simulink model "powerwindow02"  (Simulink 6.0)
settings: Solver=ode23t  StartTime=0.0  StopTime=inf  FixedStep=1e-4  RelTol=1e-2
libraries: powerlib2 x22, mblibv1 x18, simulink x6
settings Model: Creator=The MathWorks Inc.  LastModifiedBy=batserve  ExtModeAutoUpdateStatusClock=off
settings DataIOCC: SignalLoggingName=sigsOut
settings OptimizationCC: BooleanDataType=off
settings DebuggingCC: CheckExecutionContextPreStartOutputMsg=on  CheckExecutionContextRuntimeOutputMsg=on  SolverPrmCheckMsg=none
settings HardwareCC: TargetUnknown=on
settings SimMechanicsCC: VisOnUpdateDiagram=on

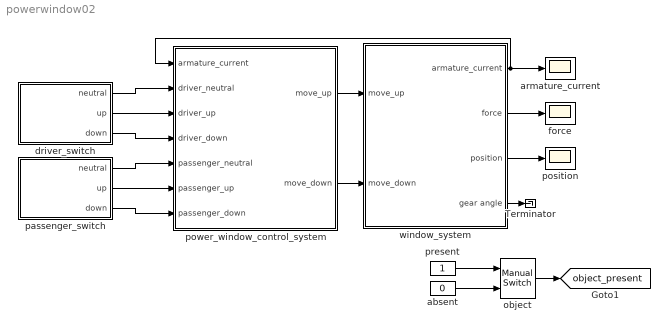
== system powerwindow02 ==
  Terminator : Terminator
  absent : Constant  Value=0
  armature_current : Scope
      settings: DataFormat=Array
  driver_switch : Subsystem  PropExecContextAcrossSSBoundary=on
  force : Scope
      settings: DataFormat=Array
  object : simulink/Signal Routing/Manual Switch  sw=1  action=0
  passenger_switch : Subsystem  PropExecContextAcrossSSBoundary=on
  position : Scope
      settings: YMin=-0.05  YMax=0.5  DataFormat=Array
  power_window_control_system : Subsystem  PropExecContextAcrossSSBoundary=on
  present : Constant
  window_system : Subsystem  PropExecContextAcrossSSBoundary=on
  tag scope: object_present=global
  wires:
  driver_switch/1(neutral) -> power_window_control_system/2(driver_neutral)
  driver_switch/2(up) -> power_window_control_system/3(driver_up)
  driver_switch/3(down) -> power_window_control_system/4(driver_down)
  passenger_switch/1(neutral) -> power_window_control_system/5(passenger_neutral)
  passenger_switch/2(up) -> power_window_control_system/6(passenger_up)
  passenger_switch/3(down) -> power_window_control_system/7(passenger_down)
  power_window_control_system/1(move_up) -> window_system/1(move_up)
  power_window_control_system/2(move_down) -> window_system/2(move_down)
  window_system/1(armature_current) -> armature_current/1, power_window_control_system/1(armature_current)
  window_system/2(force) -> force/1
  window_system/3(position) -> position/1
  present/1 -> object/1
  absent/1 -> object/2
  object/1 -> [object_present]
  window_system/4(gear angle) -> Terminator/1

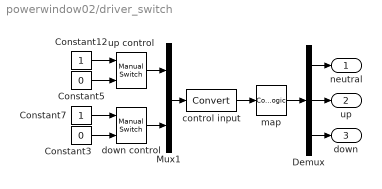
== system powerwindow02/driver_switch ==
  Constant12 : Constant
  Constant3 : Constant  Value=0
  Constant5 : Constant  Value=0
  Constant7 : Constant
  Demux : Demux  Outputs=3
  Mux1 : Mux  Inputs=2
  control input : DataTypeConversion  OutDataTypeMode=boolean  SaturateOnIntegerOverflow=on  RndMeth=Zero
  down control : simulink/Signal Routing/Manual Switch  sw=0  action=0
  map : CombinatorialLogic  TruthTable=[1 0 0;0 0 1;0 1 0;1 0 0]
  up control : simulink/Signal Routing/Manual Switch  sw=0  action=0
  neutral : Outport
  up : Outport  Port=2
  down : Outport  Port=3
  wires:
  control input/1 -> map/1
  Constant12/1 -> up control/1
  Constant5/1 -> up control/2
  Constant7/1 -> down control/1
  Constant3/1 -> down control/2
  down control/1 -> Mux1/2
  Mux1/1 -> control input/1
  up control/1 -> Mux1/1
  map/1 -> Demux/1
  Demux/1 -> neutral/1
  Demux/2 -> up/1
  Demux/3 -> down/1

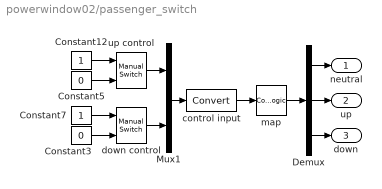
== system powerwindow02/passenger_switch ==
  Constant12 : Constant
  Constant3 : Constant  Value=0
  Constant5 : Constant  Value=0
  Constant7 : Constant
  Demux : Demux  Outputs=3
  Mux1 : Mux  Inputs=2
  control input : DataTypeConversion  OutDataTypeMode=boolean  SaturateOnIntegerOverflow=on  RndMeth=Zero
  down control : simulink/Signal Routing/Manual Switch  sw=0  action=0
  map : CombinatorialLogic  TruthTable=[1 0 0;0 0 1;0 1 0;1 0 0]
  up control : simulink/Signal Routing/Manual Switch  sw=0  action=0
  neutral : Outport
  up : Outport  Port=2
  down : Outport  Port=3
  wires:
  Demux/3 -> down/1
  Demux/2 -> up/1
  Demux/1 -> neutral/1
  map/1 -> Demux/1
  up control/1 -> Mux1/1
  Mux1/1 -> control input/1
  down control/1 -> Mux1/2
  Constant3/1 -> down control/2
  Constant7/1 -> down control/1
  Constant5/1 -> up control/2
  Constant12/1 -> up control/1
  control input/1 -> map/1

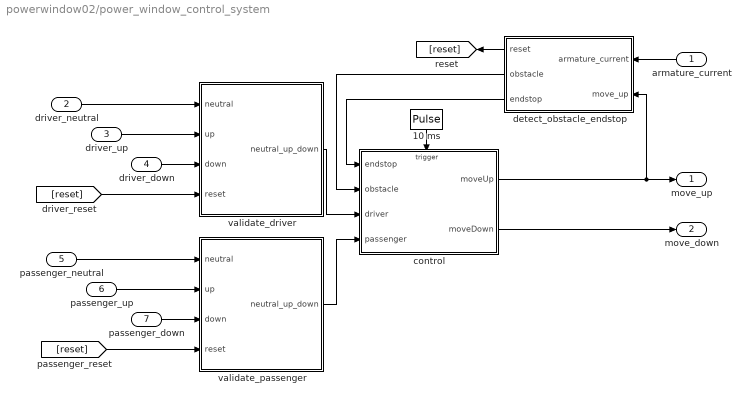
== system powerwindow02/power_window_control_system ==
  armature_current : Inport  Orientation=left  Port=1  LatchInput=off
  driver_neutral : Inport  Port=2  LatchInput=off
  driver_up : Inport  Port=3  LatchInput=off
  driver_down : Inport  Port=4  LatchInput=off
  passenger_neutral : Inport  Port=5  LatchInput=off
  passenger_up : Inport  Port=6  LatchInput=off
  passenger_down : Inport  Port=7  LatchInput=off
  10 ms : DiscretePulseGenerator  Orientation=down  SampleTime=10e-3
  control : Stateflow chart  TreatAsAtomicUnit=on  PropExecContextAcrossSSBoundary=on
  detect_obstacle_endstop : Subsystem  Orientation=left  PropExecContextAcrossSSBoundary=on
  validate_driver : Subsystem  PropExecContextAcrossSSBoundary=on
  validate_passenger : Subsystem  PropExecContextAcrossSSBoundary=on
  move_up : Outport
  move_down : Outport  Port=2
  wires:
  detect_obstacle_endstop/2(obstacle) -> control/2(obstacle)
  detect_obstacle_endstop/3(endstop) -> control/1(endstop)
  detect_obstacle_endstop/1(reset) -> [reset]
  armature_current/1 -> detect_obstacle_endstop/1(armature_current)
  10 ms/1 -> control/Trigger
  control/1(moveUp) -> detect_obstacle_endstop/2(move_up), move_up/1
  control/2(moveDown) -> move_down/1
  driver_neutral/1 -> validate_driver/1(neutral)
  driver_up/1 -> validate_driver/2(up)
  driver_down/1 -> validate_driver/3(down)
  [reset] -> validate_driver/4(reset)
  passenger_neutral/1 -> validate_passenger/1(neutral)
  passenger_up/1 -> validate_passenger/2(up)
  passenger_down/1 -> validate_passenger/3(down)
  [reset] -> validate_passenger/4(reset)
  validate_driver/1(neutral_up_down) -> control/3(driver)
  validate_passenger/1(neutral_up_down) -> control/4(passenger)

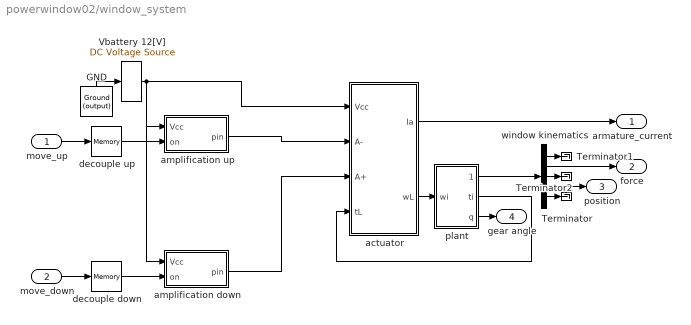
== system powerwindow02/window_system ==
  move_up : Inport  Port=1  LatchInput=off
  move_down : Inport  Port=2  LatchInput=off
  GND : powerlib2/Connectors/Ground (output)  Tag=PoWeRsYsTeMbLoCk  Orientation=up  PSBOutputType=1
  Terminator : Terminator
  Terminator1 : Terminator
  Terminator2 : Terminator
  Vbattery 12[V] : powerlib2/Electrical Sources/DC Voltage Source  Tag=PoWeRsYsTeMbLoCk  V=12  mesure=None  PSBOutputType=1
  actuator : Subsystem  PropExecContextAcrossSSBoundary=on
  amplification down : Subsystem  PropExecContextAcrossSSBoundary=on
  amplification up : Subsystem  PropExecContextAcrossSSBoundary=on
  decouple down : Memory
  decouple up : Memory
  plant : Subsystem  PropExecContextAcrossSSBoundary=on
  window kinematics : Demux  Outputs=[1,1,2,1,4]
  armature_current : Outport
  force : Outport  Port=2
  position : Outport  Port=3
  gear angle : Outport  Port=4
  wires:
  decouple down/1 -> amplification down/2(on)
  decouple up/1 -> amplification up/2(on)
  plant/3(q) -> gear angle/1
  GND/1 -> Vbattery 12[V]/1
  Vbattery 12[V]/1 -> amplification up/1(Vcc), amplification down/1(Vcc), actuator/1(Vcc)
  amplification up/1(pin) -> actuator/2(A-)
  amplification down/1(pin) -> actuator/3(A+)
  actuator/2(wL) -> plant/1(wi)
  plant/2(ti) -> actuator/4(tL)
  plant/1("F, x, v") -> window kinematics/1
  actuator/1(Ia) -> armature_current/1
  move_up/1 -> decouple up/1
  move_down/1 -> decouple down/1
  window kinematics/2 -> force/1
  window kinematics/1 -> Terminator1/1
  window kinematics/4 -> position/1
  window kinematics/5 -> Terminator/1
  window kinematics/3 -> Terminator2/1

== system powerwindow02/power_window_control_system/detect_obstacle_endstop ==
  armature_current : Inport  Port=1  LatchInput=off
  move_up : Inport  Port=2  LatchInput=off
  detect_endstop : Subsystem  PropExecContextAcrossSSBoundary=on
  detect_obstacle : Subsystem  PropExecContextAcrossSSBoundary=on
  either : Logic  Operator=OR
  process_current : Subsystem  PropExecContextAcrossSSBoundary=on
  reset : Outport
  obstacle : Outport  Port=2
  endstop : Outport  Port=3
  wires:
  armature_current/1 -> process_current/1(raw_current)
  detect_obstacle/1(obstacle) -> either/1, obstacle/1
  detect_endstop/1(endstop) -> endstop/1, either/2
  either/1 -> reset/1
  move_up/1 -> detect_obstacle/1(move_up)
  process_current/1(processed_current) -> detect_obstacle/2(armature_current), detect_endstop/1(armature_current)

== system powerwindow02/power_window_control_system/validate_driver ==
  neutral : Inport  Port=1  LatchInput=off
  up : Inport  Port=2  LatchInput=off
  down : Inport  Port=3  LatchInput=off
  reset : Inport  Port=4  LatchInput=off
  Mux : Mux  Inputs=3
  check_down : Subsystem  PropExecContextAcrossSSBoundary=on
  check_up : Subsystem  PropExecContextAcrossSSBoundary=on
  mutually_exclusive : Subsystem  PropExecContextAcrossSSBoundary=on
  neutral_up_down : Outport
  wires:
  Mux/1 -> neutral_up_down/1
  reset/1 -> [reset]
  [reset] -> check_down/2(reset)
  [reset] -> check_up/2(reset)
  check_up/1(checked_action) -> mutually_exclusive/2(up)
  neutral/1 -> mutually_exclusive/1(neutral)
  up/1 -> check_up/1(action)
  down/1 -> check_down/1(action)
  mutually_exclusive/1(validated_neutral) -> Mux/1
  mutually_exclusive/2(validated_up) -> Mux/2
  mutually_exclusive/3(validated_down) -> Mux/3
  check_down/1(checked_action) -> mutually_exclusive/3(down)

== system powerwindow02/power_window_control_system/validate_passenger ==
  neutral : Inport  Port=1  LatchInput=off
  up : Inport  Port=2  LatchInput=off
  down : Inport  Port=3  LatchInput=off
  reset : Inport  Port=4  LatchInput=off
  Mux : Mux  Inputs=3
  check_down : Subsystem  PropExecContextAcrossSSBoundary=on
  check_up : Subsystem  PropExecContextAcrossSSBoundary=on
  mutually_exclusive : Subsystem  PropExecContextAcrossSSBoundary=on
  neutral_up_down : Outport
  wires:
  Mux/1 -> neutral_up_down/1
  reset/1 -> [reset]
  [reset] -> check_down/2(reset)
  [reset] -> check_up/2(reset)
  check_up/1(checked_action) -> mutually_exclusive/2(up)
  neutral/1 -> mutually_exclusive/1(neutral)
  up/1 -> check_up/1(action)
  down/1 -> check_down/1(action)
  mutually_exclusive/1(validated_neutral) -> Mux/1
  mutually_exclusive/2(validated_up) -> Mux/2
  mutually_exclusive/3(validated_down) -> Mux/3
  check_down/1(checked_action) -> mutually_exclusive/3(down)

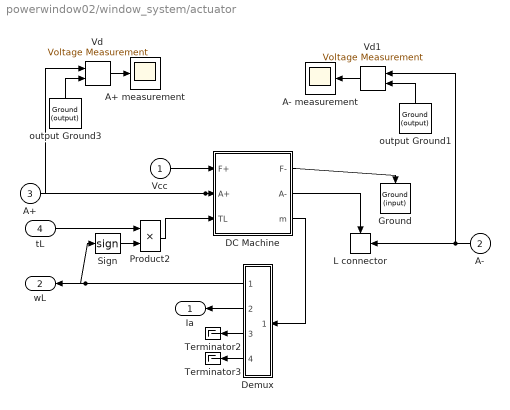
== system powerwindow02/window_system/actuator ==
  Vcc : Inport  Port=1  LatchInput=off
  A- : Inport  Orientation=left  Port=2  LatchInput=off
  A+ : Inport  Port=3  LatchInput=off
  tL : Inport  Port=4  LatchInput=off
  A+ measurement : Scope
      settings: TimeRange=0.12  YMin=11.8065  YMax=11.8095  SaveName=ScopeData2
  A- measurement : Scope
      settings: TimeRange=0.12  YMin=11.9431  YMax=11.9433  SaveName=ScopeData3
  DC Machine : Subsystem  PropExecContextAcrossSSBoundary=on  mask(DC machine){RLa=[0.15  0.036], RLf=[1.5 3], Laf=1, J=0.085, Bm=5, Tf=0, w0=0, PSBOutputType=110}
      mask prompts: RLa "Armature resistance and inductance [Ra (ohms) La (H) ]"; RLf "Field resistance and inductance [Rf (ohms) Lf (H) ]"; Laf "Field-armature mutual inductance Laf (H) :"; J "Total inertia J (kg.m^2)"; Bm "Viscous friction coefficient Bm (N.m.s)"; Tf "Coulomb friction torque Tf (N.m)"; w0 "Initial speed (rad/s) :"; PSBOutputType "Output type"
      mask help:
      | This block implements a separately excited DC machine. Access is provided  to the field connections so that the machine can be used as a shunt-connected or a series-connected  DC machine.
      |
      | Input 1 and output 1 : positive and negative armature terminals
      | Input 2 and output 2 : positive and negative field terminals
      | Input 3    : Load torque
      | Output 3 : Simulink measurement output [ w Ia If Te ]
      mask init:
      | Ra=RLa(1); La=RLa(2);
      | Rf=RLf(1); Lf=RLf(2);
      mask Help: web(psbhelp)
      mask Display: plot(-80,-80,80,80,[0,9,18,24,29,30,29,24,18,9,0,-9,-18,-24,-29,-30,-29,-24,-18,-9,0],[30,29,24,18,9,0,-9,-18,-24,-29,-30,-29,-24,-18,-9,0,9,18,24,29,30],[-29,-35,-35,-29],[-8,-8,8,8],[29,35,35,29],[-8,-8,8,8],[-35,-55],[0,0],[35,55],[0,0],[-78,-50,-50,-49,-45,-39,-33,-26,-21,-18,-17,-19,-22,-22,-26,-27,-25,-22,-16,-9,-3,2,6,6,4,1,1,-3,-4,-2,2,7,14,20,26,29,30,28,24,24,21,20,21,25,31,37,44,49,50,50,50,78]*.7,[58,58,57.2,49.2,42.8,38.8,38,39.6,44.4,51.6,59.6,67.6,72.4,72.4,65.2,57.2,49.2,42.8,38.8,38,39.6,44.4,51.6,59.6,67.6,72.4,72.4,65.2,57.2,49.2,42.8,38.8,38,39.6,44.4,51.6,59.6,67.6,72.4,72.4,65.2,57.2,49.2,42.8,38.8,38,39.6,44.4,51.6,58,58,58]*.6+15 );
  Demux : Subsystem  Orientation=left  PropExecContextAcrossSSBoundary=on
  Ground : powerlib2/Connectors/Ground (input)  Tag=PoWeRsYsTeMbLoCk  Orientation=down
  L connector : powerlib2/Connectors/L connector  Tag=PoWeRsYsTeMbLoCk  Orientation=left
  Product2 : Product  SaturateOnIntegerOverflow=on  InputSameDT=on
  Sign : Signum
  Terminator2 : Terminator
  Terminator3 : Terminator
  Vd : powerlib2/Measurements/Voltage Measurement  Tag=PoWeRsYsTeMmEaSuReMeNt  PhasorSimulation=off  OutputType=Magnitude  PSBOutputType=0  PSBequivalent=0
  Vd1 : powerlib2/Measurements/Voltage Measurement  Tag=PoWeRsYsTeMmEaSuReMeNt  Orientation=left  PhasorSimulation=off  OutputType=Magnitude  PSBOutputType=0  PSBequivalent=0
  output Ground1 : powerlib2/Connectors/Ground (output)  Tag=PoWeRsYsTeMbLoCk  Orientation=up  PSBOutputType=1
  output Ground3 : powerlib2/Connectors/Ground (output)  Tag=PoWeRsYsTeMbLoCk  Orientation=up  PSBOutputType=1
  Ia : Outport  Orientation=left
  wL : Outport  Orientation=left  Port=2
  wires:
  A+/1 -> DC Machine/2(A+), Vd/1
  Demux/4(Te) -> Terminator3/1
  Demux/3(If) -> Terminator2/1
  DC Machine/3(m) -> Demux/1(m)
  Demux/1(wm) -> Sign/1, wL/1
  Sign/1 -> Product2/2
  Product2/1 -> DC Machine/3(TL)
  tL/1 -> Product2/1
  Demux/2(Ia) -> Ia/1
  DC Machine/1(F-) -> Ground/1
  Vcc/1 -> DC Machine/1(F+)
  A-/1 -> Vd1/1, L connector/1
  DC Machine/2(A-) -> L connector/Enable
  output Ground3/1 -> Vd/2
  Vd/1 -> A+ measurement/1
  output Ground1/1 -> Vd1/2
  Vd1/1 -> A- measurement/1

== system powerwindow02/window_system/amplification down ==
  Vcc : Inport  Port=1  LatchInput=off
  on : Inport  Port=2  LatchInput=off
  Logical Operator : Logic  Operator=NOT
  Terminator1 : Terminator
  Terminator2 : Terminator
  connector : powerlib2/Connectors/T connector  Tag=PoWeRsYsTeMbLoCk  PSBOutputType=1
  output Ground1 : powerlib2/Connectors/Ground (output)  Tag=PoWeRsYsTeMbLoCk  Orientation=up  PSBOutputType=1
  up switch : powerlib2/Power Electronics/Ideal Switch  Tag=PoWeRsYsTeMbLoCk  Ron=0.01  Lon=0  IC=0  Rs=1000000  Cs=inf  PSBOutputType=10
  up switch1 : powerlib2/Power Electronics/Ideal Switch  Tag=PoWeRsYsTeMbLoCk  Ron=0.01  Lon=0  IC=0  Rs=1000000  Cs=inf  PSBOutputType=10
  pin : Outport  InitialOutput=0
  wires:
  on/1 -> Logical Operator/1, up switch/2
  Vcc/1 -> up switch/1
  up switch/2 -> Terminator1/1
  output Ground1/1 -> up switch1/1
  up switch1/2 -> Terminator2/1
  up switch/1 -> connector/1
  connector/1 -> pin/1
  up switch1/1 -> connector/Enable
  Logical Operator/1 -> up switch1/2

== system powerwindow02/window_system/amplification up ==
  Vcc : Inport  Port=1  LatchInput=off
  on : Inport  Port=2  LatchInput=off
  Logical Operator : Logic  Operator=NOT
  Terminator1 : Terminator
  Terminator2 : Terminator
  connector : powerlib2/Connectors/T connector  Tag=PoWeRsYsTeMbLoCk  PSBOutputType=1
  output Ground1 : powerlib2/Connectors/Ground (output)  Tag=PoWeRsYsTeMbLoCk  Orientation=up  PSBOutputType=1
  up switch : powerlib2/Power Electronics/Ideal Switch  Tag=PoWeRsYsTeMbLoCk  Ron=0.01  Lon=0  IC=0  Rs=1000000  Cs=inf  PSBOutputType=10
  up switch1 : powerlib2/Power Electronics/Ideal Switch  Tag=PoWeRsYsTeMbLoCk  Ron=0.01  Lon=0  IC=0  Rs=1000000  Cs=inf  PSBOutputType=10
  pin : Outport  InitialOutput=0
  wires:
  on/1 -> Logical Operator/1, up switch/2
  Vcc/1 -> up switch/1
  up switch/2 -> Terminator1/1
  output Ground1/1 -> up switch1/1
  up switch1/2 -> Terminator2/1
  up switch/1 -> connector/1
  connector/1 -> pin/1
  up switch1/1 -> connector/Enable
  Logical Operator/1 -> up switch1/2

== system powerwindow02/window_system/plant ==
  wi : Inport  Port=1  LatchInput=off
  Demux1 : Demux  Outputs=[4, 1, 2, 1, 1]
  Terminator : Terminator
  Terminator1 : Terminator
  Terminator2 : Terminator
  object : Subsystem  PropExecContextAcrossSSBoundary=on
  window : Subsystem  PropExecContextAcrossSSBoundary=on
  "F, x, v" : Outport
  ti : Outport  Port=2
  q : Outport  Port=3
  wires:
  window/2(ti) -> ti/1
  wi/1 -> window/1(wi)
  object/1(torque) -> window/2(Fx)
  window/3(q) -> q/1
  Demux1/4 -> object/2(velocity)
  Demux1/2 -> object/1(position)
  Demux1/1 -> Terminator/1
  Demux1/3 -> Terminator1/1
  Demux1/5 -> Terminator2/1
  window/1(F,d,v) -> Demux1/1, "F, x, v"/1

== system powerwindow02/power_window_control_system/detect_obstacle_endstop/detect_endstop ==
  armature_current : Inport  Port=1  LatchInput=off
  Constant6 : Constant  Value=15
  current_limit : RelationalOperator  Operator=>  InputSameDT=on
  passenger control : DataTypeConversion  OutDataTypeMode=boolean  SaturateOnIntegerOverflow=on  RndMeth=Zero
  endstop : Outport
  wires:
  passenger control/1 -> endstop/1
  current_limit/1 -> passenger control/1
  armature_current/1 -> current_limit/1
  Constant6/1 -> current_limit/2

== system powerwindow02/power_window_control_system/detect_obstacle_endstop/detect_obstacle ==
  move_up : Inport  Orientation=left  Port=1  LatchInput=off
  armature_current : Inport  Port=2  LatchInput=off
  10 ms1 : DiscretePulseGenerator  Orientation=down  SampleTime=10e-3
  Constant1 : Constant  Value=1.7
  Product : Product  Orientation=up  SaturateOnIntegerOverflow=on  InputSameDT=on
  break dependency : UnitDelay  Orientation=left  SampleTime=0.01
  delay_detection : Stateflow chart  Orientation=left  TreatAsAtomicUnit=on  PropExecContextAcrossSSBoundary=on
  object : RelationalOperator  Operator=>  InputSameDT=on
  passenger control : DataTypeConversion  Orientation=up  OutDataTypeMode=boolean  SaturateOnIntegerOverflow=on  RndMeth=Zero
  obstacle : Outport  Orientation=up
  wires:
  passenger control/1 -> obstacle/1
  break dependency/1 -> delay_detection/1(move_up)
  10 ms1/1 -> delay_detection/Trigger
  Product/1 -> passenger control/1
  move_up/1 -> break dependency/1
  armature_current/1 -> object/1
  delay_detection/1(detect) -> Product/2
  object/1 -> Product/1
  Constant1/1 -> object/2

== system powerwindow02/power_window_control_system/detect_obstacle_endstop/process_current ==
  raw_current : Inport  Port=1  LatchInput=off
  Abs : Abs  SaturateOnIntegerOverflow=on
  processed_current : Outport
  wires:
  raw_current/1 -> Abs/1
  Abs/1 -> processed_current/1

== system powerwindow02/power_window_control_system/validate_driver/check_down ==
  action : Inport  Port=1  LatchInput=off
  reset : Inport  Port=2  LatchInput=off
  allow_action : Logic
  overrule : Logic  Operator=NOT
  checked_action : Outport
  wires:
  reset/1 -> overrule/1
  allow_action/1 -> checked_action/1
  action/1 -> allow_action/1
  overrule/1 -> allow_action/2

== system powerwindow02/power_window_control_system/validate_driver/check_up ==
  action : Inport  Port=1  LatchInput=off
  reset : Inport  Port=2  LatchInput=off
  allow_action : Logic
  overrule : Logic  Operator=NOT
  checked_action : Outport
  wires:
  overrule/1 -> allow_action/2
  action/1 -> allow_action/1
  allow_action/1 -> checked_action/1
  reset/1 -> overrule/1

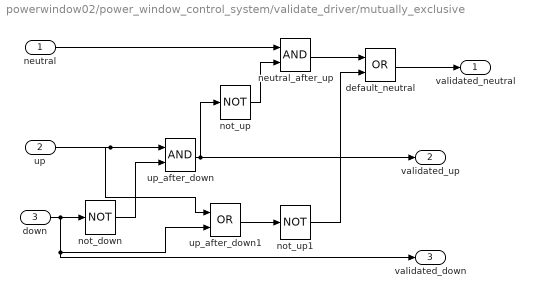
== system powerwindow02/power_window_control_system/validate_driver/mutually_exclusive ==
  neutral : Inport  Port=1  LatchInput=off
  up : Inport  Port=2  LatchInput=off
  down : Inport  Port=3  LatchInput=off
  default_neutral : Logic  Operator=OR
  neutral_after_up : Logic
  not_down : Logic  Operator=NOT
  not_up : Logic  Operator=NOT
  not_up1 : Logic  Operator=NOT
  up_after_down : Logic
  up_after_down1 : Logic  Operator=OR
  validated_neutral : Outport
  validated_up : Outport  Port=2
  validated_down : Outport  Port=3
  wires:
  not_down/1 -> up_after_down/2
  up_after_down/1 -> not_up/1, validated_up/1
  not_up/1 -> neutral_after_up/2
  down/1 -> not_down/1, up_after_down1/2, validated_down/1
  neutral/1 -> neutral_after_up/1
  up/1 -> up_after_down/1, up_after_down1/1
  up_after_down1/1 -> not_up1/1
  neutral_after_up/1 -> default_neutral/1
  default_neutral/1 -> validated_neutral/1
  not_up1/1 -> default_neutral/2

== system powerwindow02/power_window_control_system/validate_passenger/check_down ==
  action : Inport  Port=1  LatchInput=off
  reset : Inport  Port=2  LatchInput=off
  allow_action : Logic
  overrule : Logic  Operator=NOT
  checked_action : Outport
  wires:
  reset/1 -> overrule/1
  allow_action/1 -> checked_action/1
  action/1 -> allow_action/1
  overrule/1 -> allow_action/2

== system powerwindow02/power_window_control_system/validate_passenger/check_up ==
  action : Inport  Port=1  LatchInput=off
  reset : Inport  Port=2  LatchInput=off
  allow_action : Logic
  overrule : Logic  Operator=NOT
  checked_action : Outport
  wires:
  overrule/1 -> allow_action/2
  action/1 -> allow_action/1
  allow_action/1 -> checked_action/1
  reset/1 -> overrule/1

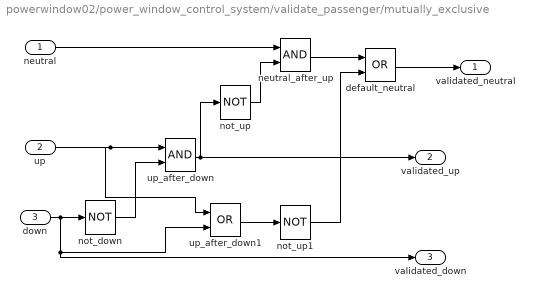
== system powerwindow02/power_window_control_system/validate_passenger/mutually_exclusive ==
  neutral : Inport  Port=1  LatchInput=off
  up : Inport  Port=2  LatchInput=off
  down : Inport  Port=3  LatchInput=off
  default_neutral : Logic  Operator=OR
  neutral_after_up : Logic
  not_down : Logic  Operator=NOT
  not_up : Logic  Operator=NOT
  not_up1 : Logic  Operator=NOT
  up_after_down : Logic
  up_after_down1 : Logic  Operator=OR
  validated_neutral : Outport
  validated_up : Outport  Port=2
  validated_down : Outport  Port=3
  wires:
  not_down/1 -> up_after_down/2
  up_after_down/1 -> not_up/1, validated_up/1
  not_up/1 -> neutral_after_up/2
  down/1 -> not_down/1, up_after_down1/2, validated_down/1
  neutral/1 -> neutral_after_up/1
  up/1 -> up_after_down/1, up_after_down1/1
  up_after_down1/1 -> not_up1/1
  neutral_after_up/1 -> default_neutral/1
  default_neutral/1 -> validated_neutral/1
  not_up1/1 -> default_neutral/2

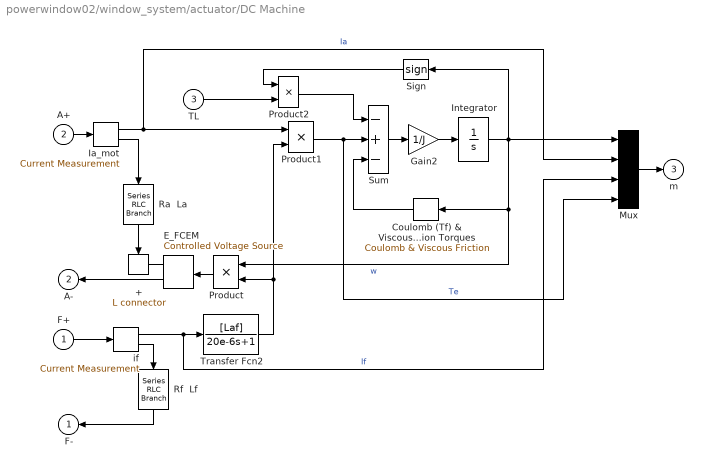
== system powerwindow02/window_system/actuator/DC Machine ==
  F+ : Inport  Port=1  LatchInput=off
  A+ : Inport  Port=2  LatchInput=off
  TL : Inport  Port=3  LatchInput=off
  + : powerlib2/Connectors/L connector  Tag=PoWeRsYsTeMbLoCk  Orientation=down
  Coulomb (Tf) & Viscous ( Bm*w)  Friction Torques : simulink/Discontinuities/Coulomb & Viscous Friction  Orientation=left  offset=Tf  gain=Bm
  E_FCEM : powerlib2/Electrical Sources/Controlled Voltage Source  Tag=PoWeRsYsTeMbLoCk  Orientation=left  initsrc=on  srctyp=AC  iv=0  iph=0  ifreq=0  mesure=None  PSBOutputType=11
  Gain2 : Gain  Gain=1/J  SaturateOnIntegerOverflow=on
  Ia_mot : powerlib2/Measurements/Current Measurement  Tag=PoWeRsYsTeMmEaSuReMeNt  PhasorSimulation=off  OutputType=Magnitude  PSBOutputType=01  PSBequivalent=0
  Integrator : Integrator  InitialCondition=w0
  Mux : Mux
  Product : Product  Orientation=left  SaturateOnIntegerOverflow=on  InputSameDT=on
  Product1 : Product  SaturateOnIntegerOverflow=on  InputSameDT=on
  Product2 : Product  SaturateOnIntegerOverflow=on  InputSameDT=on
  Ra  La : powerlib2/Elements/Series RLC Branch  Tag=PoWeRsYsTeMbLoCk  Orientation=down  a=Ra  b=La  c=inf  mesure=None  PSBOutputType=1
  Rf  Lf : powerlib2/Elements/Series RLC Branch  Tag=PoWeRsYsTeMbLoCk  Orientation=down  a=Rf  b=Lf  c=inf  mesure=None  PSBOutputType=1
  Sign : Signum  Orientation=left
  Sum : Sum  Inputs=-+-  SaturateOnIntegerOverflow=on  InputSameDT=on
  Transfer Fcn2 : TransferFcn  Numerator=[Laf]  Denominator=[20e-6 1]
  if : powerlib2/Measurements/Current Measurement  Tag=PoWeRsYsTeMmEaSuReMeNt  PhasorSimulation=off  OutputType=Magnitude  PSBOutputType=01  PSBequivalent=0
  F- : Outport  Orientation=left  InitialOutput=0
  A- : Outport  Orientation=left  Port=2  InitialOutput=0
  m : Outport  Port=3  InitialOutput=0
  wires:
  Coulomb (Tf) & Viscous ( Bm*w)  Friction Torques/1 -> Sum/3
  Transfer Fcn2/1 -> Product/2, Product1/2
  Mux/1 -> m/1
  Product1/1 -> Mux/4, Sum/2  "Te"
  Product/1 -> E_FCEM/1
  Integrator/1 -> Sign/1, Mux/1, Product/1, Coulomb (Tf) & Viscous ( Bm*w)  Friction Torques/1  "w"
  Gain2/1 -> Integrator/1
  Sum/1 -> Gain2/1
  Sign/1 -> Product2/1
  TL/1 -> Product2/2
  Product2/1 -> Sum/1
  if/1 -> Mux/3, Transfer Fcn2/1  "If"
  Ia_mot/1 -> Mux/2, Product1/1  "Ia"
  Rf  Lf/1 -> F-/1
  E_FCEM/2 -> A-/1
  E_FCEM/1 -> +/Enable
  if/2 -> Rf  Lf/1
  F+/1 -> if/1
  Ra  La/1 -> +/1
  Ia_mot/2 -> Ra  La/1
  A+/1 -> Ia_mot/1

== system powerwindow02/window_system/actuator/Demux ==
  m : Inport  Port=1  LatchInput=off
  Demux : Demux
  wm : Outport
  Ia : Outport  Port=2
  If : Outport  Port=3
  Te : Outport  Port=4
  wires:
  Demux/4 -> Te/1
  Demux/3 -> If/1
  m/1 -> Demux/1
  Demux/2 -> Ia/1
  Demux/1 -> wm/1

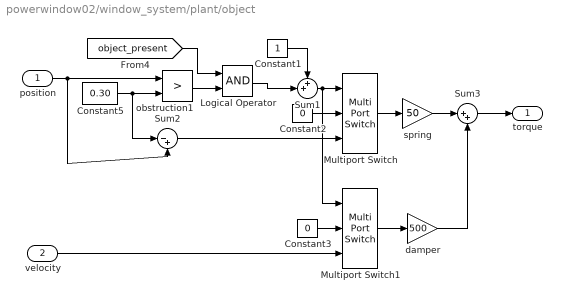
== system powerwindow02/window_system/plant/object ==
  position : Inport  Port=1  LatchInput=off
  velocity : Inport  Port=2  LatchInput=off
  Constant1 : Constant
  Constant2 : Constant  Value=0
  Constant3 : Constant  Value=0
  Constant5 : Constant  Value=0.30
  Logical Operator : Logic
  Multiport Switch : MultiPortSwitch  Inputs=2  InputSameDT=on
  Multiport Switch1 : MultiPortSwitch  Inputs=2  InputSameDT=on
  Sum1 : Sum  Inputs=++|  SaturateOnIntegerOverflow=on  InputSameDT=on
  Sum2 : Sum  Inputs=|-+  SaturateOnIntegerOverflow=on  InputSameDT=on
  Sum3 : Sum  Inputs=|++  SaturateOnIntegerOverflow=on  InputSameDT=on
  damper : Gain  Gain=500  SaturateOnIntegerOverflow=on
  obstruction1 : RelationalOperator  Operator=>  InputSameDT=on
  spring : Gain  Gain=50  SaturateOnIntegerOverflow=on
  torque : Outport
  wires:
  [object_present] -> Logical Operator/1
  Logical Operator/1 -> Sum1/2
  obstruction1/1 -> Logical Operator/2
  Multiport Switch1/1 -> damper/1
  velocity/1 -> Multiport Switch1/3
  Constant3/1 -> Multiport Switch1/2
  Multiport Switch/1 -> spring/1
  position/1 -> Sum2/2, obstruction1/1
  Constant1/1 -> Sum1/1
  Sum2/1 -> Multiport Switch/3
  Constant2/1 -> Multiport Switch/2
  Sum1/1 -> Multiport Switch1/1, Multiport Switch/1
  Constant5/1 -> Sum2/1, obstruction1/2
  damper/1 -> Sum3/2
  Sum3/1 -> torque/1
  spring/1 -> Sum3/1

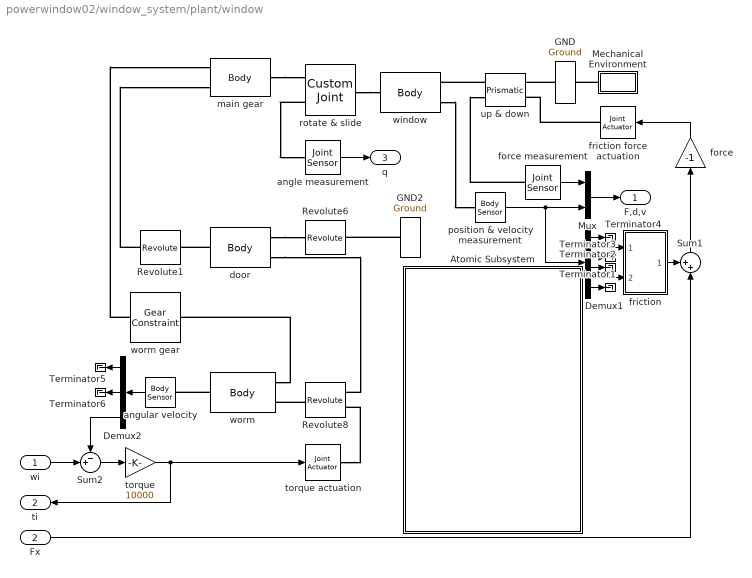
== system powerwindow02/window_system/plant/window ==
  wi : Inport  Port=1  LatchInput=off
  Fx : Inport  Port=2  LatchInput=off
  Atomic Subsystem : Subsystem  TreatAsAtomicUnit=on  PropExecContextAcrossSSBoundary=on
      mask Display: image(imread('pw_window1c.jpg'))
  Demux1 : Demux  Outputs=6
  Demux2 : Demux  Orientation=left  Outputs=3
  GND : mblibv1/Bodies/Ground  Orientation=left  Opaque=on  LeftPortType=env  RightPortType=workingframe  PhysicalDomain=Mechanical  DialogClass=GroundBlock  CoordPosition=[10 0 0]  CoordPositionUnits=cm  StateVectorMgrId=-1  MachineId=[0 0]  ShowEnvPort=on
  GND2 : mblibv1/Bodies/Ground  Orientation=left  Opaque=on  LeftPortType=env  RightPortType=workingframe  PhysicalDomain=Mechanical  DialogClass=GroundBlock  CoordPosition=[0 0 0]  CoordPositionUnits=m  StateVectorMgrId=-1  MachineId=[0 0]  ShowEnvPort=off
  Mechanical Environment : Subsystem  Tag=Factory ground  Orientation=left  DialogController=MECH.DialogSource  PropExecContextAcrossSSBoundary=on  Opaque=on  mask(Mechanical){PortType=env, PhysicalDomain=Mechanical, ClassName=Environment, DialogTemplateClass=MECH.MachineEnvironment, SyncWhenCopied=off, Gravity=[0 0 0], GravityUnits=m/s^2, GravityAsSignal=off, Dimensionality=3D Only, AnalysisType=Forward dynamics, LinearAssemblyTolerance=1e-3, LinearAssemblyToleranceUnits=m, AngularAssemblyTolerance=1e-3, AngularAssemblyToleranceUnits=rad, ConstraintSolverType=Stabilizing, ConstraintRelTolerance=1e-4, ConstraintAbsTolerance=1e-4, UseRobustSingularityHandling=off, StatePerturbationType=Fixed, PerturbationSize=1e-5, VisualizeMachine=on}
      mask help: Defines the mechanical simulation environment for the machine to which the block is connected: gravity, dimensionality, analysis mode, constraint solver type, tolerances, linearization, and visualization.
      mask init:
      | mech_environment_block('MaskInitialization', gcbh);
      settings: CopyFcn=mech_environment_block('CopyFcn', gcbh);
      mask Help: web(mech_help('environment'))
      mask StyleString: edit,edit,edit,edit,edit,edit,popup(km/s^2|m/s^2|cm/s^2|mm/s^2|mi/s^2|ft/s^2|in/s^2),checkbox,popup(2D Only|3D Only|Auto-detect),popup(Forward dynamics|Inverse dynamics|Kinematics|Trimming),edit,popup(km|m|cm|mm|mi|ft|in),edit,popup(deg|rad),popup(Stabilizing|Tolerancing|Machine precision),edit,edit,checkbox,popup(Adaptive|Fixed),edit,checkbox
      mask Display: disp('Env')
  Mux : Mux  Inputs=2
  Revolute1 : mblibv1/Joints/Revolute  Tag=Factory generic  Description=Mechanical Blockset  Orientation=left  PhysicalDomain=mechanical  SubClassName=Unknown  LeftPortType=blob  RightPortType=blob  LConnTagsString=__newl0  RConnTagsString=__newr0  NumSAPorts=0  CutJoint=off  MarkAsCut=off  Primitives=revolute  PrimitiveProps=R1$WORLD$[0 0 1]$revolute  DialogClass=JointBlock
  Revolute6 : mblibv1/Joints/Revolute  Tag=Factory generic  Description=Mechanical Blockset  Orientation=left  PhysicalDomain=mechanical  SubClassName=Unknown  LeftPortType=blob  RightPortType=blob  LConnTagsString=__newl0  RConnTagsString=__newr0  NumSAPorts=0  CutJoint=off  MarkAsCut=off  Primitives=revolute  PrimitiveProps=R1$WORLD$[1 0 0]$revolute  DialogClass=JointBlock
  Revolute8 : mblibv1/Joints/Revolute  Tag=Factory generic  Description=Mechanical Blockset  Orientation=left  PhysicalDomain=mechanical  SubClassName=Unknown  LeftPortType=blob  RightPortType=blob  LConnTagsString=__newl0|SA1  RConnTagsString=__newr0  NumSAPorts=1  CutJoint=off  MarkAsCut=off  Primitives=revolute  PrimitiveProps=R1$WORLD$[0 0 1]$revolute  DialogClass=JointBlock
  Sum1 : Sum  Orientation=up  Inputs=++|  SaturateOnIntegerOverflow=on  InputSameDT=on
  Sum2 : Sum  Inputs=-+|  SaturateOnIntegerOverflow=on  InputSameDT=on
  Terminator{1..6} (6 alike) : Terminator
  angle measurement : mblibv1/Sensors &  Actuators/Joint Sensor  Description=Mechanical Blockset  Opaque=on  PhysicalDomain=Mechanical  PortType=blob  Muxed=on  Pose=off  Angle=on  AngleUnits=rad  ArcVelocity=off  ArcVelocityUnits=deg/s  ArcAcceleration=off  ArcAccelerationUnits=deg/s^2  CoordPosition=off  CoordPositionUnits=m  Velocity=off  VelocityUnits=m/s  Acceleration=off  AccelerationUnits=m/s^2  Quaternion=on  QuaternionDT=off  QuaternionDDT=off  QuaternionUnits=off  OutputVector=[ 1 ]  ActiveIO=off  Width=1  DialogClass=MechanicalSensorBlock  Primitive=R1  Force=off  ForceUnits=N  Torque=off  TorqueUnits=N-m  ReferenceFrame=Absolute (INERTIAL)  ReactionSensedSide=Base  ReactionReferenceFrame=Absolute (World)  ReactionForce=off  ReactionForceUnits=N  ReactionMoment=off  ReactionMomentUnits=N-m
  angular velocity : mblibv1/Sensors &  Actuators/Body Sensor  Description=Mechanical Blockset  Orientation=left  Opaque=on  PhysicalDomain=Mechanical  PortType=blob  Muxed=on  Pose=off  Angle=on  AngleUnits=deg  ArcVelocity=on  ArcVelocityUnits=rad/s  ArcAcceleration=off  ArcAccelerationUnits=deg/s^2  CoordPosition=off  CoordPositionUnits=m  Velocity=off  VelocityUnits=m/s  Acceleration=off  AccelerationUnits=m/s^2  Quaternion=on  QuaternionDT=off  QuaternionDDT=off  QuaternionUnits=off  OutputVector=[ 3 ]  ActiveIO=off  Width=1  DialogClass=MechanicalSensorBlock  ReferenceFrame=Absolute (World)
  door : mblibv1/Bodies/Body  Tag=Factory generic  Description=Mechanical Blockset  Orientation=left  PhysicalDomain=mechanical  SubClassName=Unknown  LeftPortType=workingframe  RightPortType=workingframe  LConnTagsString=CS3|CG  RConnTagsString=CS1  DialogClass=MechanicalBodyBlock  Mass=1  MassUnits=kg  InertiaUnits=kg*m^2  Inertia=eye(3)  Shape=Cylinder  ShapeDims=[1 1]  ShapeUnits=m  ShapeUse=false  Density=1  DensityUnits=kg/m^3  DensityUse=false  CG=Left$CG$[0 0 0]$WORLD$WORLD$cm$[0 0 0]$Euler X-Y-Z$deg$WORLD$true  WorkingFrames=Left$CS3$[0 0 0]$CG$CG$cm$[0 0 0]$Euler X-Y-Z$deg$WORLD$true#Right$CS1$[17 0 0]$CG$CG$cm$[0 0 0]$Euler X-Y-Z$deg$WORLD$true
  force : Gain  Orientation=up  Gain=-1  SaturateOnIntegerOverflow=on
  force measurement : mblibv1/Sensors &  Actuators/Joint Sensor  Description=Mechanical Blockset  Opaque=on  PhysicalDomain=Mechanical  PortType=blob  Muxed=on  Pose=off  Angle=on  AngleUnits=deg  ArcVelocity=off  ArcVelocityUnits=deg/s  ArcAcceleration=off  ArcAccelerationUnits=deg/s^2  CoordPosition=off  CoordPositionUnits=m  Velocity=off  VelocityUnits=m/s  Acceleration=off  AccelerationUnits=m/s^2  Quaternion=on  QuaternionDT=off  QuaternionDDT=off  QuaternionUnits=off  OutputVector=[ 3 ]  ActiveIO=off  Width=1  DialogClass=MechanicalSensorBlock  Primitive=P1  Force=off  ForceUnits=N  Torque=off  TorqueUnits=N-m  ReferenceFrame=Absolute (INERTIAL)  ReactionSensedSide=Base  ReactionReferenceFrame=Absolute (World)  ReactionForce=on  ReactionForceUnits=N  ReactionMoment=off  ReactionMomentUnits=N-m
  friction : Subsystem  PropExecContextAcrossSSBoundary=on
  friction force actuation : mblibv1/Sensors &  Actuators/Joint Actuator  Description=Mechanical Blockset  Orientation=left  Opaque=on  PhysicalDomain=Mechanical  PortType=blob  ActuationStyle=Force  AngleUnits=deg  ArcVelocityUnits=deg/s  ArcAccelerationUnits=deg/s^2  CoordPositionUnits=m  VelocityUnits=m/s  AccelerationUnits=m/s^2  ForceUnits=N  TorqueUnits=N-m  ActiveIO=off  Width=1  DialogClass=MechanicalActuatorBlock  Primitive=P1  ReferenceFrame=Absolute (INERTIAL)
  main gear : mblibv1/Bodies/Body  Tag=Factory generic  Description=Mechanical Blockset  PhysicalDomain=mechanical  SubClassName=Unknown  LeftPortType=workingframe  RightPortType=workingframe  LConnTagsString=CS3|CG  RConnTagsString=CS1  DialogClass=MechanicalBodyBlock  Mass=2  MassUnits=kg  InertiaUnits=kg*m^2  Inertia=eye(3)  Shape=Cylinder  ShapeDims=[1 1]  ShapeUnits=m  ShapeUse=false  Density=1  DensityUnits=kg/m^3  DensityUse=false  CG=Left$CG$[17 0 0]$WORLD$WORLD$cm$[0 0 0]$Euler X-Y-Z$deg$WORLD$true  WorkingFrames=Left$CS3$[0 0 0]$CG$CG$cm$[0 0 0]$Euler X-Y-Z$deg$WORLD$true#Right$CS1$[60 0 0]$CG$CG$cm$[0 0 0]$Euler X-Y-Z$deg$WORLD$true
  position & velocity measurement : mblibv1/Sensors &  Actuators/Body Sensor  Description=Mechanical Blockset  Opaque=on  PhysicalDomain=Mechanical  PortType=blob  Muxed=on  Pose=off  Angle=on  AngleUnits=deg  ArcVelocity=off  ArcVelocityUnits=deg/s  ArcAcceleration=off  ArcAccelerationUnits=deg/s^2  CoordPosition=on  CoordPositionUnits=m  Velocity=on  VelocityUnits=m/s  Acceleration=off  AccelerationUnits=m/s^2  Quaternion=on  QuaternionDT=off  QuaternionDDT=off  QuaternionUnits=off  OutputVector=[ 3 3 ]  ActiveIO=off  Width=1  DialogClass=MechanicalSensorBlock  ReferenceFrame=Absolute (World)
  rotate & slide : mblibv1/Joints/Custom Joint  Tag=Factory generic  Description=Mechanical Blockset  PhysicalDomain=mechanical  SubClassName=custom_joint  LeftPortType=blob  RightPortType=blob  LConnTagsString=__newl0|SA1  RConnTagsString=__newr0  NumSAPorts=1  CutJoint=off  MarkAsCut=off  Primitives=revolute_prismatic  PrimitiveProps=R1$Base$[0 0 1]$revolute#P1$Follower$[1 0 0]$prismatic  DialogClass=JointBlock
  torque : Gain  Gain=10000  SaturateOnIntegerOverflow=on
  torque actuation : mblibv1/Sensors &  Actuators/Joint Actuator  Description=Mechanical Blockset  Opaque=on  PhysicalDomain=Mechanical  PortType=blob  ActuationStyle=Force  AngleUnits=deg  ArcVelocityUnits=deg/s  ArcAccelerationUnits=deg/s^2  CoordPositionUnits=m  VelocityUnits=m/s  AccelerationUnits=m/s^2  ForceUnits=N  TorqueUnits=N-m  ActiveIO=off  Width=1  DialogClass=MechanicalActuatorBlock  Primitive=R1  ReferenceFrame=Absolute (INERTIAL)
  up & down : mblibv1/Joints/Prismatic  Tag=Factory generic  Description=Mechanical Blockset  Orientation=left  PhysicalDomain=mechanical  SubClassName=Unknown  LeftPortType=blob  RightPortType=blob  LConnTagsString=__newl0|SA1  RConnTagsString=__newr0|SA1  NumSAPorts=2  CutJoint=on  MarkAsCut=off  Primitives=prismatic  PrimitiveProps=P1$WORLD$[0 1 0]$prismatic  DialogClass=JointBlock
  window : mblibv1/Bodies/Body  Tag=Factory generic  Description=Mechanical Blockset  PhysicalDomain=mechanical  SubClassName=Unknown  LeftPortType=workingframe  RightPortType=workingframe  LConnTagsString=CS1  RConnTagsString=CS2|CS3  DialogClass=MechanicalBodyBlock  Mass=5  MassUnits=kg  InertiaUnits=kg*m^2  Inertia=eye(3)  Shape=Cylinder  ShapeDims=[1 1]  ShapeUnits=m  ShapeUse=false  Density=1  DensityUnits=kg/m^3  DensityUse=false  CG=Left$CG$[10 0 0]$WORLD$WORLD$cm$[0 0 0]$Euler X-Y-Z$deg$WORLD$false  WorkingFrames=Left$CS1$[0 0 0]$CG$CG$cm$[0 0 0]$Euler X-Y-Z$deg$WORLD$true#Right$CS2$[0 0 0]$CG$CG$cm$[0 0 0]$Euler X-Y-Z$deg$WORLD$true#Right$CS3$[-15 0 0]$CG$CG$cm$[0 0 0]$Euler X-Y-Z$deg$WORLD$true
  worm : mblibv1/Bodies/Body  Tag=Factory generic  Description=Mechanical Blockset  Orientation=left  PhysicalDomain=mechanical  SubClassName=Unknown  LeftPortType=workingframe  RightPortType=workingframe  LConnTagsString=CS3|CS4  RConnTagsString=CG  DialogClass=MechanicalBodyBlock  Mass=0.5  MassUnits=kg  InertiaUnits=kg*m^2  Inertia=eye(3)  Shape=Cylinder  ShapeDims=[1 1]  ShapeUnits=m  ShapeUse=false  Density=1  DensityUnits=kg/m^3  DensityUse=false  CG=Right$CG$[0 0 0]$WORLD$WORLD$cm$[0 0 0]$Euler X-Y-Z$deg$WORLD$true  WorkingFrames=Left$CS3$[0 0 0]$CG$CG$cm$[0 0 0]$Euler X-Y-Z$deg$WORLD$true#Left$CS4$[0 0 0]$CG$CG$cm$[0 0 0]$Euler X-Y-Z$deg$WORLD$true
  worm gear : mblibv1/Constraints &  Drivers/Gear Constraint  Tag=Factory generic  Description=Mechanical Blockset  Orientation=left  PhysicalDomain=mechanical  SubClassName=Unknown  LeftPortType=blob  RightPortType=blob  LConnTagsString=__newl0  RConnTagsString=__newr0  DialogClass=GearConstraint  NumSAPorts=0  BaseRadius=2  BaseRadiusUnits=cm  FollowerRadius=15  FollowerRadiusUnits=cm
  F,d,v : Outport
  ti : Outport  Orientation=left  Port=2
  q : Outport  Port=3
  wires:
  angle measurement/1 -> q/1
  Mux/1 -> F,d,v/1
  force measurement/1 -> Mux/1
  position & velocity measurement/1 -> Mux/2, Demux1/1
  Demux1/2 -> friction/1(position)
  Demux1/5 -> friction/2(velocity)
  torque/1 -> ti/1, torque actuation/1
  Sum2/1 -> torque/1
  angular velocity/1 -> Demux2/1
  Demux2/3 -> Sum2/1
  wi/1 -> Sum2/2
  Fx/1 -> Sum1/2
  friction/1(torque) -> Sum1/1
  Sum1/1 -> force/1
  force/1 -> friction force actuation/1
  Demux1/6 -> Terminator1/1
  Demux1/4 -> Terminator2/1
  Demux1/3 -> Terminator3/1
  Demux1/1 -> Terminator4/1
  Demux2/1 -> Terminator5/1
  Demux2/2 -> Terminator6/1
  connections:
  rotate & slide/LConn2 -- angle measurement/LConn1
  force measurement/LConn1 -- up & down/RConn2
  friction force actuation/RConn1 -- up & down/LConn2
  Revolute8/RConn1 -- worm/LConn2
  worm/LConn1 -- worm gear/LConn1
  door/RConn1 -- Revolute1/LConn1
  Revolute1/RConn1 -- main gear/LConn2
  worm gear/RConn1 -- main gear/LConn1
  door/LConn1 -- Revolute6/RConn1
  GND2/RConn1 -- Revolute6/LConn1
  torque actuation/RConn1 -- Revolute8/LConn2
  door/LConn2 -- Revolute8/LConn1
  main gear/RConn1 -- rotate & slide/LConn1
  rotate & slide/RConn1 -- window/LConn1
  window/RConn2 -- position & velocity measurement/LConn1
  GND/RConn1 -- up & down/LConn1
  up & down/RConn1 -- window/RConn1
  worm/RConn1 -- angular velocity/LConn1
  Mechanical Environment/RConn1 -- GND/LConn1

== system powerwindow02/window_system/plant/window/Atomic Subsystem ==

== system powerwindow02/window_system/plant/window/Mechanical Environment ==
  SOURCE_BLOCK : Constant  Value=Gravity
  TERM_BLOCK : Terminator
  out : PMIOPort  Port=1  Side=Right
  tag scope: sim_mech_taga61585042e8c20b9=global
  wires:
  SOURCE_BLOCK/1 -> [sim_mech_taga61585042e8c20b9]
  [sim_mech_taga61585042e8c20b9] -> TERM_BLOCK/1

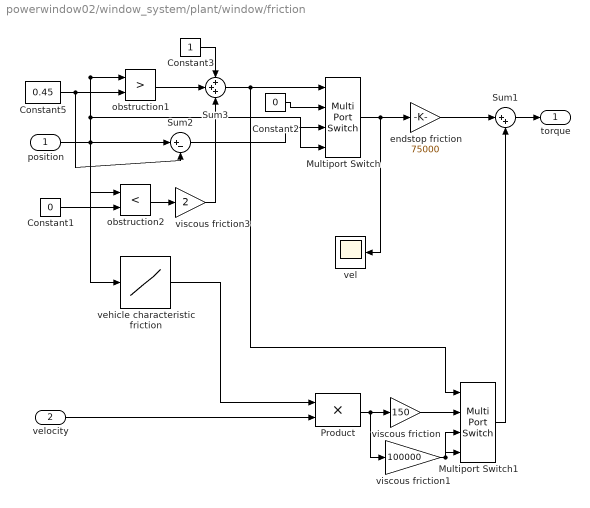
== system powerwindow02/window_system/plant/window/friction ==
  position : Inport  Port=1  LatchInput=off
  velocity : Inport  Port=2  LatchInput=off
  Constant1 : Constant  Value=0
  Constant2 : Constant  Value=0
  Constant3 : Constant
  Constant5 : Constant  Value=0.45
  Multiport Switch : MultiPortSwitch  Inputs=3  InputSameDT=on
  Multiport Switch1 : MultiPortSwitch  Inputs=3  InputSameDT=on
  Product : Product  SaturateOnIntegerOverflow=on  InputSameDT=on
  Sum1 : Sum  Inputs=|++  SaturateOnIntegerOverflow=on  InputSameDT=on
  Sum2 : Sum  Inputs=|+-  SaturateOnIntegerOverflow=on  InputSameDT=on
  Sum3 : Sum  Inputs=+++  SaturateOnIntegerOverflow=on  InputSameDT=on
  endstop friction : Gain  Gain=75000  SaturateOnIntegerOverflow=on
  obstruction1 : RelationalOperator  Operator=>  InputSameDT=on
  obstruction2 : RelationalOperator  Operator=<  InputSameDT=on
  vehicle characteristic friction : Lookup  DialogController=Simulink.DDGSource  InputValues=[0 2.5 10 11.5 14 24 30 31 35 47 50]  OutputValues=[1.15 1.2 1.05 1.1 1.05 1 1.1 1 0.95 0.9 0.95]  SaturateOnIntegerOverflow=on
  vel : Scope
      settings: YMin=-1  YMax=1  SaveName=ScopeData6
  viscous friction3 : Gain  Gain=2  SaturateOnIntegerOverflow=on
  viscous friction : Gain  Gain=150  SaturateOnIntegerOverflow=on
  viscous friction1 : Gain  Gain=100000  SaturateOnIntegerOverflow=on
  torque : Outport
  wires:
  Sum1/1 -> torque/1
  velocity/1 -> Product/2
  position/1 -> obstruction1/1, obstruction2/1, Multiport Switch/4, Sum2/1, vehicle characteristic friction/1
  Constant5/1 -> obstruction1/2, Sum2/2
  Constant1/1 -> obstruction2/2
  endstop friction/1 -> Sum1/1
  Constant2/1 -> Multiport Switch/2
  Sum2/1 -> Multiport Switch/3
  obstruction2/1 -> viscous friction3/1
  obstruction1/1 -> Sum3/2
  viscous friction3/1 -> Sum3/3
  Constant3/1 -> Sum3/1
  Sum3/1 -> Multiport Switch/1, Multiport Switch1/1
  Multiport Switch/1 -> endstop friction/1, vel/1
  Product/1 -> viscous friction/1, viscous friction1/1
  vehicle characteristic friction/1 -> Product/1
  viscous friction/1 -> Multiport Switch1/2
  Multiport Switch1/1 -> Sum1/2
  viscous friction1/1 -> Multiport Switch1/3, Multiport Switch1/4

== stateflow chart power_window_control_system/control ==
  settings: executeAtInitialization=1
  state emergencyDown
    entry:
    moveUp = 0;
    moveDown = 1;
  state safe
    state driverUp
      entry: moveUp = 1;
      exit: moveUp = 0;
      state iniDriverUp
      state DriverUp
      state autoDriverUp
      iniDriverUp -> (junction 26) : after(100,ticks)
      (junction 26) -> DriverUp
      (junction 26) -> autoDriverUp : [driver[1]]
    state driverDown
      entry: moveDown = 1;
      exit: moveDown = 0;
      state iniDriverDown
      state DriverDown
      state autoDriverDown
      iniDriverDown -> (junction 25) : after(100,ticks)
      (junction 25) -> autoDriverDown : [driver[1]]
      (junction 25) -> DriverDown
    state driverNeutral
      entry:
      moveUp = 0;
      moveDown = 0;
      state passengerneutral
        entry:
        moveUp = 0;
        moveDown = 0;
      state passengerUp
        entry: moveUp = 1;
        exit: moveUp = 0;
        state iniPassengerUp
        state PassengerUp
        state autoPassengerUp
        (junction 24) -> PassengerUp
        (junction 24) -> autoPassengerUp : [passenger[1]]
        iniPassengerUp -> (junction 24) : after(100,ticks)
      state passengerDown
        entry: moveDown = 1;
        exit: moveDown = 0;
        state iniPassengerDown
        state passengerDown
        state autoPassengerDown
        (junction 23) -> autoPassengerDown : [passenger[1]]
        iniPassengerDown -> (junction 23) : after(100,ticks)
        (junction 23) -> safe.driverNeutral.passengerDown.passengerDown
      safe.driverNeutral.passengerDown.passengerDown -> passengerneutral : [passenger[1]]
      safe.driverNeutral.passengerDown -> passengerneutral : [endstop]
      PassengerUp -> passengerneutral : [passenger[1]]
      passengerUp -> passengerneutral : [endstop]
      passengerneutral -> iniPassengerDown : [passenger[3]]
      passengerneutral -> iniPassengerUp : [passenger[2]]
      safe.driverNeutral.passengerDown -> PassengerUp : [passenger[2]]
      passengerUp -> safe.driverNeutral.passengerDown.passengerDown : [passenger[3]]
      (default) -> passengerneutral
    driverNeutral -> iniDriverDown : [driver[3]]
    driverUp -> DriverDown : [driver[3]]
    driverDown -> DriverUp : [driver[2]]
    driverNeutral -> iniDriverUp : [driver[2]]
    DriverDown -> driverNeutral : [driver[1]]
    DriverUp -> driverNeutral : [driver[1]]
    driverDown -> driverNeutral : [endstop]
    driverUp -> driverNeutral : [endstop]
    (default) -> driverNeutral
  emergencyDown -> passengerneutral : [endstop | after(100,ticks)]
  safe -> emergencyDown : [obstacle]
  (default) -> safe
  data: moveUp output double; moveDown output double; endstop input boolean; obstacle input boolean; driver input boolean size=3; passenger input boolean size=3
  events: ticks input EITHER_EDGE_EVENT

== stateflow chart power_window_control_system/detect_obstacle_endstop/detect_obstacle/delay_detection ==
  settings: executeAtInitialization=1
  state detect
  state off
  state hold
  (default) -> off
  off -> hold : [move_up]
  detect -> off : [~move_up]
  hold -> detect : [after(100,ticks)]
  hold -> off : [~move_up]
  data: detect output State; move_up input boolean
  events: ticks input EITHER_EDGE_EVENT
